simulink model "CAVFinal"  (R2025b)
settings: Solver=VariableStepAuto  StartTime=0.0  StopTime=20  RelTol=1e-3
undefined symbols (not defined in the file or in its folder): kd_head, kd_lat, ki_lat, kp_ff, kp_head, kp_lat
libraries: autolibshared x1
settings Model: SimulationMode=accelerator  Creator=moddi  LastModifiedBy=anith

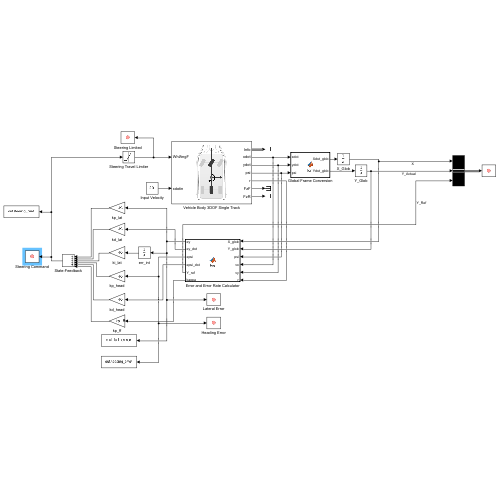
[thumbnail: Simulink's stored preview of the top-level diagram]
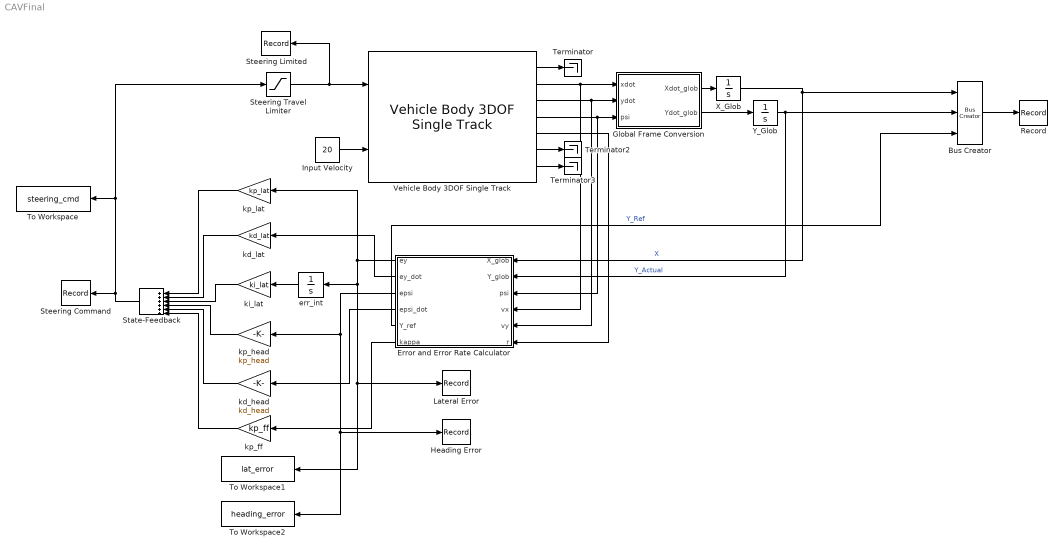
== system CAVFinal ==
  Bus Creator : BusCreator  Inputs=3
  Error and Error Rate Calculator : MATLAB Function  TreatAsAtomicUnit=on
  Global Frame Conversion : MATLAB Function  TreatAsAtomicUnit=on
  Heading Error : Record  NumPorts=1.0  FileSettingsInternal="{\"entries\":[{\"content\":{\"excelSettings\":{\"content\":{},\"type\":\"Streamout.ExcelSettings\"},\"parquetSettings\":{\"content\":{},\"type\":\"Streamout.ParquetSettings\"}},\"type\":\"Streamout.FileSettingStorage\",\"uuid\":\"\"}],\"packageUris\":[\"http:\\/\\/schema.mathworks.com\\/mf0\\/streamout_blocks\\/R2020a\"],\"version\":\"1.0\"}"  FrameSettings=0  Layout=[1 1]  SignalsInternal="{\"entries\":[{\"content\":{\"signals\":[{\"content\":{\"blockPath\":[],\"dimensions\":[1],\"domain\":\"\",\"lineColor\":\"#edb120\",\"lineWidth\":2,\"plots\":[ 1 ],\"port\":1,\"sid\":[\"\"],\"signalID\":1,\"signalName\":\"Error and Error Rate Calculator:3\"},\"type\":\"RecordBlkView.Signal\",\"uuid\":\"\"}]},\"type\":\"RecordBlkView.InputSignals\",\"uuid\":\"\"}],\"packageUris\":[\"http:\\/\\/schema.mathworks.com\\/mf0\\/streamout_blocks\\/R2020a\"],\"version\":\"1.0\"}"  VisualizationBindings="{\"sparklinesplugin\":{\"info\":[{\"bindingParametersList\":[],\"subplotID\":1}]}}"
  Input Velocity : Constant  Value=20
  Lateral Error : Record  NumPorts=1.0  FileSettingsInternal="{\"entries\":[{\"content\":{\"excelSettings\":{\"content\":{},\"type\":\"Streamout.ExcelSettings\"},\"parquetSettings\":{\"content\":{},\"type\":\"Streamout.ParquetSettings\"}},\"type\":\"Streamout.FileSettingStorage\",\"uuid\":\"\"}],\"packageUris\":[\"http:\\/\\/schema.mathworks.com\\/mf0\\/streamout_blocks\\/R2020a\"],\"version\":\"1.0\"}"  FrameSettings=0  Layout=[1 1]  SignalsInternal="{\"entries\":[{\"content\":{\"signals\":[{\"content\":{\"blockPath\":[],\"dimensions\":[1],\"domain\":\"\",\"lineColor\":\"#0072bd\",\"lineWidth\":4,\"plots\":[ 1 ],\"port\":1,\"sid\":[\"\"],\"signalID\":1,\"signalName\":\"Error and Error Rate Calculator:1\"},\"type\":\"RecordBlkView.Signal\",\"uuid\":\"\"}]},\"type\":\"RecordBlkView.InputSignals\",\"uuid\":\"\"}],\"packageUris\":[\"http:\\/\\/schema.mathworks.com\\/mf0\\/streamout_blocks\\/R2020a\"],\"version\":\"1.0\"}"
  Record : Record  NumPorts=1.0  FileSettingsInternal="{\"entries\":[{\"content\":{\"excelSettings\":{\"content\":{},\"type\":\"Streamout.ExcelSettings\"},\"parquetSettings\":{\"content\":{},\"type\":\"Streamout.ParquetSettings\"}},\"type\":\"Streamout.FileSettingStorage\",\"uuid\":\"\"}],\"packageUris\":[\"http:\\/\\/schema.mathworks.com\\/mf0\\/streamout_blocks\\/R2020a\"],\"version\":\"1.0\"}"  FrameSettings=0  Layout=[1 1]  SignalsInternal="{\"entries\":[{\"content\":{\"signals\":[{\"content\":{\"blockPath\":[],\"dimensions\":[1],\"domain\":\"\",\"hasChildren\":true,\"lineColor\":\"#77ac30\",\"lineWidth\":2,\"port\":1,\"sid\":[\"\"],\"signalID\":1,\"signalName\":\"Bus\\nCreator\"},\"type\":\"RecordBlkView.Signal\",\"uuid\":\"\"},{\"content\":{\"blockPath\":[],\"dimensions\":[1],\"domain\":\"\",\"leafPath\":\"Bus\\nCreator.X\",\"lineColor\":\"#0072bd\",\"lineStyle\":\"DOTTED\",\"lineWidth\":2,\"parentID\":1,\"plots\":[ 1 ],\"port\":1,\"sid\":[\"\"],\"signalID\":2,\"signalName\":\"Bus\\nCreator.X\"},\"type\":\"RecordBlkView.Signal\",\"uuid\":\"\"},{\"content\":{\"blockPath\":[],\"dimensions\":[1],\"domain\":\"\",\"leafPath\":\"Bus\\nCreator.Y_Actual\",\"lineColor\":\"#139fff\",\"lineWidth\":2,\"parentID\":1,\"plots\":[ 1 ],\"port\":1,\"sid\":[\"\"],\"signalID\":3,\"signalName\":\"Bus\\nCreator.Y_Actual\"},\"type\":\"RecordBlkView.Signal\",\"uuid\":\"\"},{\"content\":{\"blockPath\":[],\"dimensions\":[1],\"domain\":\"\",\"leafPath\":\"Bus\\nCreator.Y_Ref\",\"lineColor\":\"#a2142f\",\"lineWidth\":2,\"parentID\":1,\"plots\":[ 1 ],\"port\":1,\"sid\":[\"\"],\"signalID\":4,\"signalName\":\"Bus\\nCreator.Y_Ref\"},\"type\":\"RecordBlkView.Signal\",\"uuid\":\"\"}]},\"type\":\"RecordBlkView.InputSignals\",\"uuid\":\"\"}],\"packageUris\":[\"http:\\/\\/schema.mathworks.com\\/mf0\\/streamout_blocks\\/R2020a\"],\"version\":\"1.0\"}"  VisualizationBindings="{\"xyplotplugin\":{\"info\":[{\"series\":[{\"bindingParametersList\":[{\"parameter\":\"X-Axis\",\"signalID\":2,\"signalName\":\"Bus\\nCreator.X\"},{\"parameter\":\"Y-Axis\",\"signalID\":3,\"signalName\":\"Bus\\nCreator.Y_Actual\"}],\"seriesID\":0},{\"bindingParametersList\":[{\"parameter\":\"X-Axis\",\"signalID\":2,\"signalName\":\"Bus\\nCreator.X\"},{\"parameter\":\"Y-Axis\",\"signalID\":4,\"signalName\":\"Bus\\nCreator.Y_Ref\"}],\"seriesID\":1}],\"subplotID\":1}]}}"
  State-Feedback : Sum  Inputs=|++++++
  Steering Command : Record  NumPorts=1.0  FileSettingsInternal="{\"entries\":[{\"content\":{\"excelSettings\":{\"content\":{},\"type\":\"Streamout.ExcelSettings\"},\"parquetSettings\":{\"content\":{},\"type\":\"Streamout.ParquetSettings\"}},\"type\":\"Streamout.FileSettingStorage\",\"uuid\":\"\"}],\"packageUris\":[\"http:\\/\\/schema.mathworks.com\\/mf0\\/streamout_blocks\\/R2020a\"],\"version\":\"1.0\"}"  FrameSettings=0  Layout=[1 1]  SignalsInternal="{\"entries\":[{\"content\":{\"signals\":[{\"content\":{\"blockPath\":[],\"dimensions\":[1],\"domain\":\"\",\"lineColor\":\"#edb120\",\"lineWidth\":2,\"plots\":[ 1 ],\"port\":1,\"sid\":[\"\"],\"signalID\":1,\"signalName\":\"State-Feedback\"},\"type\":\"RecordBlkView.Signal\",\"uuid\":\"\"}]},\"type\":\"RecordBlkView.InputSignals\",\"uuid\":\"\"}],\"packageUris\":[\"http:\\/\\/schema.mathworks.com\\/mf0\\/streamout_blocks\\/R2020a\"],\"version\":\"1.0\"}"  VisualizationBindings="{\"sparklinesplugin\":{\"info\":[{\"bindingParametersList\":[],\"subplotID\":1}]}}"
  Steering Limited : Record  NumPorts=1.0  FileSettingsInternal="{\"entries\":[{\"content\":{\"excelSettings\":{\"content\":{},\"type\":\"Streamout.ExcelSettings\"},\"parquetSettings\":{\"content\":{},\"type\":\"Streamout.ParquetSettings\"}},\"type\":\"Streamout.FileSettingStorage\",\"uuid\":\"\"}],\"packageUris\":[\"http:\\/\\/schema.mathworks.com\\/mf0\\/streamout_blocks\\/R2020a\"],\"version\":\"1.0\"}"  FrameSettings=0  Layout=[1 1]  SignalsInternal="{\"entries\":[{\"content\":{\"signals\":[{\"content\":{\"blockPath\":[],\"dimensions\":[1],\"domain\":\"\",\"lineColor\":\"#edb120\",\"lineWidth\":2,\"plots\":[ 1 ],\"port\":1,\"sid\":[\"\"],\"signalID\":1,\"signalName\":\"Steering Travel Limiter\"},\"type\":\"RecordBlkView.Signal\",\"uuid\":\"\"}]},\"type\":\"RecordBlkView.InputSignals\",\"uuid\":\"\"}],\"packageUris\":[\"http:\\/\\/schema.mathworks.com\\/mf0\\/streamout_blocks\\/R2020a\"],\"version\":\"1.0\"}"  VisualizationBindings="{\"sparklinesplugin\":{\"info\":[{\"bindingParametersList\":[],\"subplotID\":1}]}}"
  Steering Travel Limiter : Saturate
  Terminator : Terminator
  Terminator2 : Terminator
  Terminator3 : Terminator
  To Workspace : ToWorkspace  VariableName=steering_cmd  SampleTime=-1
      settings: Save2DSignal=2-D array (concatenate along first dimension)
  To Workspace1 : ToWorkspace  VariableName=lat_error  SampleTime=-1
      settings: Save2DSignal=2-D array (concatenate along first dimension)
  To Workspace2 : ToWorkspace  VariableName=heading_error  SampleTime=-1
      settings: Save2DSignal=2-D array (concatenate along first dimension)
  Vehicle Body 3DOF Single Track : autolibshared/Vehicle Body 3DOF Single Track  trackMode=Single (bicycle)  inputMode=External longitudinal velocity  frontSteerMode=on  rearSteerMode=off  windMode=off  muMode=off  extFMode=off  extMMode=off  htchFMode=off  htchMMode=off  extXo=off  extpsio=off  extxdoto=off  extro=off  extYo=off  extTamb=off  extydoto=off  aMode=2  NF=2  NR=2  m=1600  a=1.4  b=1.6  h=0.35  dh=1  hh=0.2  X_o=0  xdot_o=0  CalphaMode=off  sigmaMode=on  d=0  hl=0  w=[1.4,1.4]  Cy_f=50000  Cy_r=50000  sigma_f=.1  sigma_r=.1  alpha_f_brk=[-0.785, -0.628, -0.471, -0.314, -0.157, 0.000, 0.157, 0.314, 0.471, 0.628, 0.785]  Cy_f_data=[2000, 3000, 4000, 5500, 7000, 9000, 7000, 5500, 4000, 3000, 2000]  alpha_r_brk=[-0.785, -0.628, -0.471, -0.314, -0.157, 0.000, 0.157, 0.314, 0.471, 0.628, 0.785]  Cy_r_data=[2000, 3000, 4000, 5500, 7000, 9000, 7000, 5500, 4000, 3000, 2000]  Y_o=1  ydot_o=0  Izz=2000  psi_o=0  r_o=0  Af=2  Cd=.3  Cl=.1  Cpm=.1  beta_w=[0 0.01:0.01:0.3]  Cs=[0 0.01:0.01:0.3]  Cym=[0 1e-6:0.01:0.3]  Pabs=101325  Tair=273  g=9.81  mu=1  xdot_tol=.01  Fznom=5000  Fxtire_sat=7e4  Fytire_sat=7e4  longOff=0  latOff=0  vertOff=0  wrapAng=off
  X_Glob : Integrator
  Y_Glob : Integrator  InitialCondition=1
  err_int : Integrator
  kd_head : Gain  Gain=kd_head
  kd_lat : Gain  Gain=kd_lat
  ki_lat : Gain  Gain=ki_lat
  kp_ff : Gain  Gain=kp_ff
  kp_head : Gain  Gain=kp_head
  kp_lat : Gain  Gain=kp_lat
  wires:
  Input Velocity/1 -> Vehicle Body 3DOF Single Track/2
  Vehicle Body 3DOF Single Track/1 -> Terminator/1
  Vehicle Body 3DOF Single Track/6 -> Terminator2/1
  Vehicle Body 3DOF Single Track/7 -> Terminator3/1
  Vehicle Body 3DOF Single Track/2 -> Global Frame Conversion/1(xdot), Error and Error Rate Calculator/4(vx)
  Vehicle Body 3DOF Single Track/3 -> Error and Error Rate Calculator/5(vy), Global Frame Conversion/2(ydot)
  Vehicle Body 3DOF Single Track/4 -> Error and Error Rate Calculator/3(psi), Global Frame Conversion/3(psi)
  Global Frame Conversion/2(Ydot_glob) -> Y_Glob/1
  Global Frame Conversion/1(Xdot_glob) -> X_Glob/1
  X_Glob/1 -> Bus Creator/1, Error and Error Rate Calculator/1(X_glob)  "X"
  Y_Glob/1 -> Bus Creator/2, Error and Error Rate Calculator/2(Y_glob)  "Y_Actual"
  Vehicle Body 3DOF Single Track/5 -> Error and Error Rate Calculator/6(r)
  Error and Error Rate Calculator/2(ey_dot) -> kd_lat/1
  Error and Error Rate Calculator/3(epsi) -> Heading Error/1, To Workspace2/1, kp_head/1
  Error and Error Rate Calculator/4(epsi_dot) -> kd_head/1
  kd_lat/1 -> State-Feedback/2
  kp_lat/1 -> State-Feedback/1
  Steering Travel Limiter/1 -> Steering Limited/1, Vehicle Body 3DOF Single Track/1
  State-Feedback/1 -> Steering Command/1, Steering Travel Limiter/1, To Workspace/1
  Error and Error Rate Calculator/5(Y_ref) -> Bus Creator/3  "Y_Ref"
  Bus Creator/1 -> Record/1
  Error and Error Rate Calculator/1(ey) -> To Workspace1/1, Lateral Error/1, err_int/1, kp_lat/1
  ki_lat/1 -> State-Feedback/3
  kp_head/1 -> State-Feedback/4
  kd_head/1 -> State-Feedback/5
  err_int/1 -> ki_lat/1
  Error and Error Rate Calculator/6(kappa) -> kp_ff/1
  kp_ff/1 -> State-Feedback/6

== matlab function CAVFinal/Error and Error Rate Calculator ==
  data: X_glob input; ey output; Y_glob input; psi input; ey_dot output; vx input; vy input; r input; epsi output; epsi_dot output; Y_ref output; kappa output
function [ey, ey_dot, epsi, epsi_dot, Y_ref, kappa] = fcn(X_glob, Y_glob, psi, vx, vy, r)
    Wh = 2;
    X_offset = 80;
    eta = 40;

    u = (X_glob - X_offset) / eta;
    Y_ref = Wh * tanh(u) + Wh;

    slope = (Wh / eta) * (sech(u)^2);
    psi_ref = atan(slope);

    ey = Y_ref - Y_glob;
    epsi = psi_ref - psi;

    ey_dot = vy + vx * epsi;
    epsi_dot = r;

    % curvature for feedforward
    d2y = -(2 * Wh / eta^2) * sech(u)^2 * tanh(u);
    kappa = d2y / (1 + slope^2)^(3/2);
end

== matlab function CAVFinal/Global Frame Conversion ==
  data: xdot input; Xdot_glob output; ydot input; psi input; Ydot_glob output
function [Xdot_glob, Ydot_glob] = fcn(xdot, ydot, psi)
    Xdot_glob = xdot*cos(psi) - ydot*sin(psi);
    Ydot_glob = xdot*sin(psi) + ydot*cos(psi);
end
